simulink model "samphase"  (R2012b)
settings: Solver=FixedStepDiscrete  StartTime=0.0  StopTime=1  FixedStep=dt  RelTol=1e-3
InitFcn:
  | param
values from neighbouring files (symbols this model uses):
  ampl = 1    [param.m]
  atten = 0.3    [param.m]
  delay = 1    [param.m]
  dt = 0.00025    [param.m]
  freq = 1000    [param.m]
  noiseVariance = 0.5    [param.m]
  T = 0.15    [param.m]
undefined symbols (not defined in the file or in its folder): DiscIntNeverNeededParam
libraries: commchan3 x1
settings Model: Creator=mishuk  LastModifiedBy=mishuk

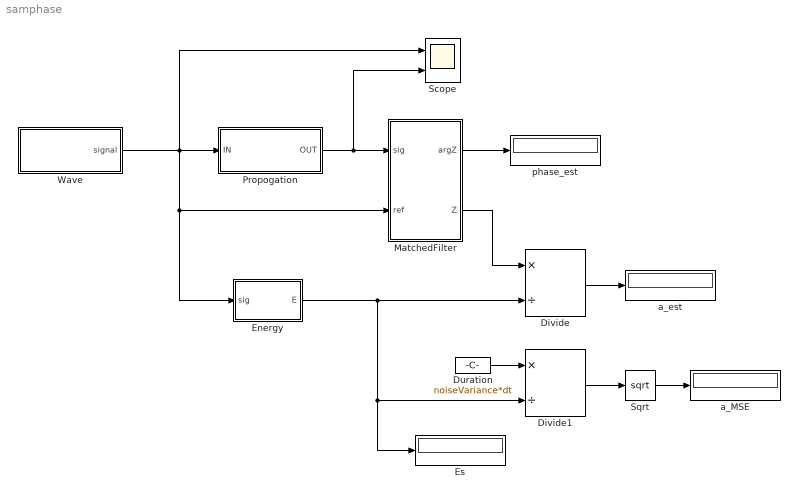
== system samphase ==
  Divide : Product  Inputs=*/
  Divide1 : Product  Inputs=*/
  Duration : Constant  Value=noiseVariance*dt
  Energy : Subsystem
  Es : Display
  MatchedFilter : Subsystem
  Propogation : Subsystem
  Scope : Scope  NumInputPorts=2
      settings: TimeRange=1  YMin=-1~-4  YMax=1~6
  Sqrt : Sqrt  SaturateOnIntegerOverflow=on
  Wave : Subsystem
  a_MSE : Display
  a_est : Display
  phase_est : Display
  wires:
  Wave/1(signal) -> Scope/1, Energy/1(sig), MatchedFilter/2(ref), Propogation/1(IN)
  Propogation/1(OUT) -> Scope/2, MatchedFilter/1(sig)
  Energy/1(E) -> Es/1, Divide1/2, Divide/2
  Divide/1 -> a_est/1
  Duration/1 -> Divide1/1
  Divide1/1 -> Sqrt/1
  Sqrt/1 -> a_MSE/1
  MatchedFilter/2(Z) -> Divide/1
  MatchedFilter/1(argZ) -> phase_est/1

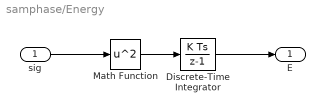
== system samphase/Energy ==
  sig : Inport
  Discrete-Time Integrator : DiscreteIntegrator  InitialCondition=1e-10  SampleTime=dt  ICPrevOutput=DiscIntNeverNeededParam  ICPrevScaledInput=DiscIntNeverNeededParam
  Math Function : Math  Operator=square  SaturateOnIntegerOverflow=on
  E : Outport
  wires:
  Discrete-Time Integrator/1 -> E/1
  sig/1 -> Math Function/1
  Math Function/1 -> Discrete-Time Integrator/1

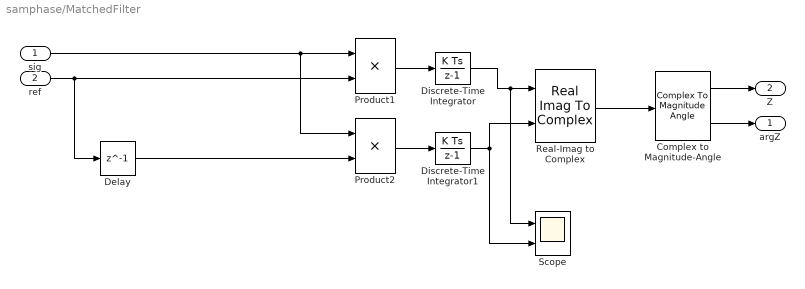
== system samphase/MatchedFilter ==
  sig : Inport
  ref : Inport  Port=2
  Complex to Magnitude-Angle : ComplexToMagnitudeAngle
  Delay : Delay  DelayLength=1  InitialCondition=0
  Discrete-Time Integrator : DiscreteIntegrator  SampleTime=dt  ICPrevOutput=DiscIntNeverNeededParam  ICPrevScaledInput=DiscIntNeverNeededParam
  Discrete-Time Integrator1 : DiscreteIntegrator  SampleTime=dt  ICPrevOutput=DiscIntNeverNeededParam  ICPrevScaledInput=DiscIntNeverNeededParam
  Product1 : Product  RndMeth=Zero
  Product2 : Product  RndMeth=Zero
  Real-Imag to Complex : RealImagToComplex
  Scope : Scope  NumInputPorts=2
      settings: TimeRange=1  YMin=-1~-4  YMax=1~6
  argZ : Outport
  Z : Outport  Port=2
  wires:
  Product1/1 -> Discrete-Time Integrator/1
  ref/1 -> Delay/1, Product1/2
  sig/1 -> Product2/1, Product1/1
  Product2/1 -> Discrete-Time Integrator1/1
  Discrete-Time Integrator/1 -> Scope/1, Real-Imag to Complex/1
  Discrete-Time Integrator1/1 -> Scope/2, Real-Imag to Complex/2
  Real-Imag to Complex/1 -> Complex to Magnitude-Angle/1
  Complex to Magnitude-Angle/2 -> argZ/1
  Complex to Magnitude-Angle/1 -> Z/1
  Delay/1 -> Product2/2

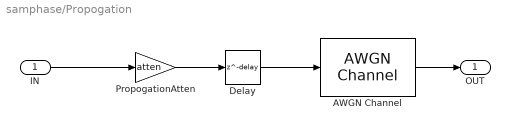
== system samphase/Propogation ==
  IN : Inport
  AWGN Channel : commchan3/AWGN Channel  InputProcessing=Columns as channels (frame based)  seed=67  noiseMode=Variance from mask  EbNodB=10  EsNodB=10  SNRdB=0  bitsPerSym=1  Ps=0.01  Tsym=1  variance=noiseVariance
  Delay : Delay  DelayLength=delay  InitialCondition=0
  PropogationAtten : Gain  Gain=atten
  OUT : Outport
  wires:
  PropogationAtten/1 -> Delay/1
  IN/1 -> PropogationAtten/1
  AWGN Channel/1 -> OUT/1
  Delay/1 -> AWGN Channel/1

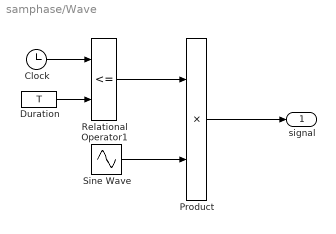
== system samphase/Wave ==
  Clock : Clock
  Duration : Constant  Value=T
  Product : Product  RndMeth=Zero
  Relational Operator1 : RelationalOperator  Operator=<=  OutDataTypeStr=boolean
  Sine Wave : Sin  Amplitude=ampl  Frequency=2*pi*freq  Phase=2*pi*rand(1)  SampleTime=dt
  signal : Outport
  wires:
  Duration/1 -> Relational Operator1/2
  Product/1 -> signal/1
  Clock/1 -> Relational Operator1/1
  Sine Wave/1 -> Product/2
  Relational Operator1/1 -> Product/1
